simulink library "Beeper"  (R2018b)
settings: Solver=VariableStepAuto  StartTime=0.0  StopTime=10.0  RelTol=1e-3
settings Model: Creator=Sjoerd  LastModifiedBy=Sjoerd

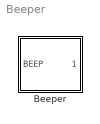
== system Beeper ==
  Beeper : Stateflow chart  TreatAsAtomicUnit=on

== stateflow chart Beeper/Beeper ==
  state Waiting
    entry:
    volume = 0
  state beep
    entry:
    volume = 50
  (default) -> Waiting
  Waiting -> beep : [BEEP]
  beep -> Waiting : after(0.5,sec)
  data: volume output int8 size=1; BEEP input boolean size=1
